simulink model "modelsCompare"  (R2023a)
settings: Solver=ode1  StartTime=0  StopTime=200  FixedStep=0.001  RelTol=1e-3  EnableMultiTasking=on
values from neighbouring files (symbols this model uses):
  B = b*L*(K_v)^2 /J_xx    (= 0.042375883612)    [advanced_model_setup.m]    (also in brusselator.m = 2.15; cycle_detection.m = img2; cycle_detection_start.m = img2; demonstrateDetections.m = 2.15)
  B1 = [-kQ, -kQ, kQ, kQ ... (first row only)    [advanced_model_setup.m]    (also in modelCompPlot.m; set_model_params.m)
  B2 = [0, 0, 0 ... (first row only)    [advanced_model_setup.m]    (also in modelCompPlot.m; set_model_params.m)
  f_p = 1.3    [advanced_model_setup.m]    (also in modelCompPlot.m)
  f_r = 0.4    [advanced_model_setup.m]    (also in modelCompPlot.m)
  f_y = 0.175    [advanced_model_setup.m]    (also in modelCompPlot.m)
  g_p = 10.5    [advanced_model_setup.m]    (also in modelCompPlot.m)
  g_r = 5.2    [advanced_model_setup.m]    (also in modelCompPlot.m)
  I_xx = 0.0522    [advanced_model_setup.m]    (also in modelCompPlot.m; set_model_params.m; solveSyms3d_2.m = evalin('base', 'I_xx'))
  I_yy = 0.0522    [advanced_model_setup.m]    (also in modelCompPlot.m; set_model_params.m; solveSyms3d_2.m = evalin('base', 'I_yy'))
  I_zz = 0.1104    [advanced_model_setup.m]    (also in modelCompPlot.m; set_model_params.m; solveSyms3d_2.m = evalin('base', 'I_zz'))
  J = (J_yy - J_zz)/J_xx    (= -1)    [advanced_model_setup.m]    (also in modelCompPlot.m)
  J_r = J_inertia/J_xx    (= 0.00108695652174)    [advanced_model_setup.m]    (also in modelCompPlot.m; solveSyms3d.m = evalin('base', 'J_r'))
  Jp = 2*Jeq_prop    (= 0.0552224595625)    [modelCompPlot.m]    (also in set_model_params.m)
  Jr = 2*Jeq_prop    (= 0.0552224595625)    [modelCompPlot.m]    (also in set_model_params.m)
  Jy = 4*Jeq_prop    (= 0.110444919125)    [modelCompPlot.m]    (also in set_model_params.m)
  K_v = 54.945    [advanced_model_setup.m]    (also in modelCompPlot.m; solveSyms3d.m = evalin('base', 'K_v'))
  Kf = 0.1188    [modelCompPlot.m]    (also in set_model_params.m)
  kfr_p = 0.4*u2line/x5line    (= 0.285774113641)    [advanced_model_setup.m]    (also in modelCompPlot.m; set_model_params.m)
  kfr_r = 0.4*u1line/x4line    (= 0.285774113641)    [advanced_model_setup.m]    (also in modelCompPlot.m; set_model_params.m)
  kfr_y = 0.4*u3line/x6line    (= 0.0880063173321)    [advanced_model_setup.m]    (also in modelCompPlot.m; set_model_params.m)
  Kt = 0.0036    [modelCompPlot.m]    (also in set_model_params.m)
  L = 0.1969    [advanced_model_setup.m]    (also in modelCompPlot.m; set_model_params.m = 0.19685)
  sigma = 0    [modelCompPlot.m]
  Y = d*(K_v)^2 /J_zz    (= 0.0032609614876)    [advanced_model_setup.m]    (also in modelCompPlot.m; solveSyms3d.m = evalin('base', 'Y'))
libraries: simulink_extras x3, dspsrcs4 x3
settings Model: ExtModeTrigDuration=10000  Creator=kille  LastModifiedBy=Jacob
settings SolverCC: PositivePriorityOrder=on  AutoInsertRateTranBlk=on
settings DataIOCC: ReturnWorkspaceOutputs=off
settings OptimizationCC: LifeSpan=inf
settings DebuggingCC: UnconnectedInputMsg=warning  UnconnectedOutputMsg=warning  UnconnectedLineMsg=warning  ArithmeticOperatorsInVariantConditions=warning
settings ModelReferenceCC: EnableRefExpFcnMdlSchedulingChecks=on
settings SFSimCC: SimUseLocalCustomCode=off  CustomCodeUndefinedFunction=UseInterfaceOnly
settings RTWCC: Description=QUARC Win64 Target  SystemTargetFile=quarc_win64.tlc  TemplateMakefile=quarc_default_tmf  RTWUseLocalCustomCode=off
settings CodeAppCC: StateflowObjectComments=on
settings STFCustomTargetCC: TargetPreCompLibLocation=C:\PROGRA~3\QUARC\lib\2016a\win64\release  UseToolchainInfoCompliant=off  SystemTargetFile=quarc_win64.tlc
settings GRTTargetCC: TargetPreCompLibLocation=C:\PROGRA~3\QUARC\lib\2016a\win64\release  ParMdlRefBuildCompliant=off  CompOptLevelCompliant=off  CombineOutputUpdateFcns=off  MatFileLogging=off  CPPClassGenCompliant=off  GRTInterface=on  UseToolchainInfoCompliant=off  ExtMode=on  ExtModeMexFile=quarc_comm
settings ConfigComp: CovMetricSettings=dswe

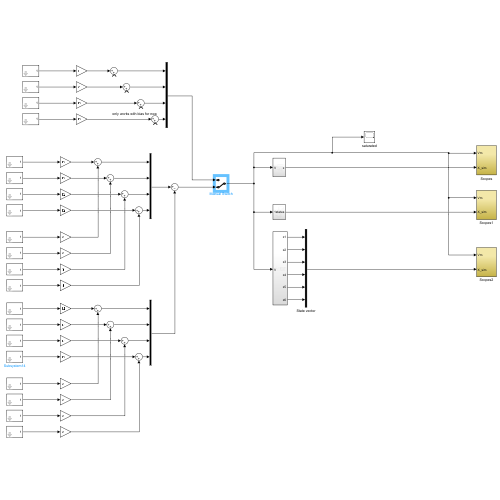
[thumbnail: Simulink's stored preview of the top-level diagram]
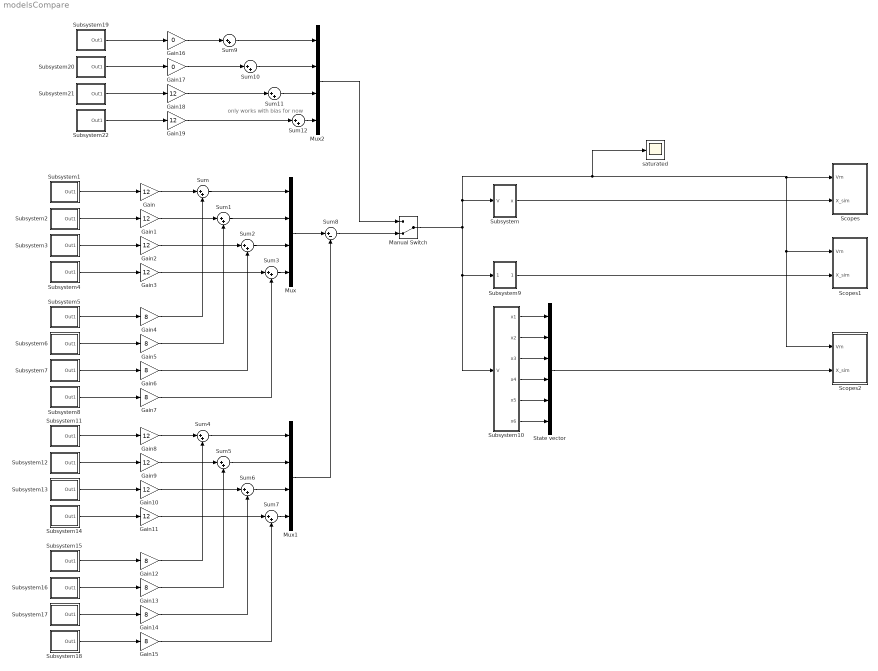
== system modelsCompare ==
  note: only works with bias for now
  Gain{,1..3,8..11,18..19} (10 alike) : Gain  Gain=12
  Gain{4..7,12..15} (8 alike) : Gain  Gain=8
  Gain16 : Gain  Gain=0
  Gain17 : Gain  Gain=0
  Manual Switch : ManualSwitch  CurrentSetting=0
  Mux : Mux
  Mux1 : Mux
  Mux2 : Mux
  Scopes : Subsystem
  Scopes1 : Subsystem
  Scopes2 : Subsystem
  State vector : Mux  Inputs=6
  Subsystem : Subsystem
  Subsystem1 : Subsystem  mask{startTime=15, duration=5, amplitude=1}
      mask prompts: startTime "Start Time"
  Subsystem10 : Subsystem
  Subsystem11 : Subsystem  mask{startTime=215, duration=5, amplitude=1}
      mask prompts: startTime "Start Time"
  Subsystem12 : Subsystem  mask{startTime=260, duration=5, amplitude=1}
      mask prompts: startTime "Start Time"
  Subsystem13 : Subsystem  mask{startTime=305, duration=5, amplitude=1}
      mask prompts: startTime "Start Time"
  Subsystem14 : Subsystem  mask{startTime=350, duration=5, amplitude=1}
      mask prompts: startTime "Start Time"
  Subsystem15 : Subsystem  mask{startTime=240, duration=5, amplitude=1}
      mask prompts: startTime "Start Time"
  Subsystem16 : Subsystem  mask{startTime=285, duration=5, amplitude=1}
      mask prompts: startTime "Start Time"
  Subsystem17 : Subsystem  mask{startTime=330, duration=5, amplitude=1}
      mask prompts: startTime "Start Time"
  Subsystem18 : Subsystem  mask{startTime=375, duration=5, amplitude=1}
      mask prompts: startTime "Start Time"
  Subsystem19 : Subsystem  mask{startTime=15, duration=5, amplitude=1}
      mask prompts: startTime "Start Time"
  Subsystem2 : Subsystem  mask{startTime=60, duration=5, amplitude=1}
      mask prompts: startTime "Start Time"
  Subsystem20 : Subsystem  mask{startTime=60, duration=5, amplitude=1}
      mask prompts: startTime "Start Time"
  Subsystem21 : Subsystem  mask{startTime=105, duration=5, amplitude=1}
      mask prompts: startTime "Start Time"
  Subsystem22 : Subsystem  mask{startTime=150, duration=5, amplitude=1}
      mask prompts: startTime "Start Time"
  Subsystem3 : Subsystem  mask{startTime=105, duration=5, amplitude=1}
      mask prompts: startTime "Start Time"
  Subsystem4 : Subsystem  mask{startTime=150, duration=5, amplitude=1}
      mask prompts: startTime "Start Time"
  Subsystem5 : Subsystem  mask{startTime=40, duration=5, amplitude=1}
      mask prompts: startTime "Start Time"
  Subsystem6 : Subsystem  mask{startTime=85, duration=5, amplitude=1}
      mask prompts: startTime "Start Time"
  Subsystem7 : Subsystem  mask{startTime=130, duration=5, amplitude=1}
      mask prompts: startTime "Start Time"
  Subsystem8 : Subsystem  mask{startTime=175, duration=5, amplitude=1}
      mask prompts: startTime "Start Time"
  Subsystem9 : Subsystem
  Sum{,1..7,9..12} (12 alike) : Sum  Inputs=|++
  Sum8 : Sum  Inputs=|+-
  saturated : Scope
  wires:
  Mux/1 -> Sum8/1
  Sum3/1 -> Mux/4
  Subsystem4/1(Out1) -> Gain3/1
  Subsystem3/1(Out1) -> Gain2/1
  Sum2/1 -> Mux/3
  Subsystem2/1(Out1) -> Gain1/1
  Sum1/1 -> Mux/2
  Subsystem1/1(Out1) -> Gain/1
  Sum/1 -> Mux/1
  Subsystem5/1(Out1) -> Gain4/1
  Subsystem6/1(Out1) -> Gain5/1
  Subsystem7/1(Out1) -> Gain6/1
  Subsystem8/1(Out1) -> Gain7/1
  Subsystem/1(x) -> Scopes/2(X_sim)
  Subsystem10/6(x6) -> State vector/6
  Subsystem10/5(x5) -> State vector/5
  Subsystem10/4(x4) -> State vector/4
  Subsystem10/3(x3) -> State vector/3
  Subsystem10/2(x2) -> State vector/2
  Subsystem10/1(x1) -> State vector/1
  State vector/1 -> Scopes2/2(X_sim)
  Subsystem9/1(states) -> Scopes1/2(X_sim)
  Gain/1 -> Sum/1
  Gain1/1 -> Sum1/1
  Gain2/1 -> Sum2/1
  Gain3/1 -> Sum3/1
  Gain4/1 -> Sum/2
  Gain5/1 -> Sum1/2
  Gain6/1 -> Sum2/2
  Gain7/1 -> Sum3/2
  Subsystem16/1(Out1) -> Gain13/1
  Subsystem14/1(Out1) -> Gain11/1
  Subsystem17/1(Out1) -> Gain14/1
  Subsystem18/1(Out1) -> Gain15/1
  Subsystem15/1(Out1) -> Gain12/1
  Sum5/1 -> Mux1/2
  Gain13/1 -> Sum5/2
  Gain12/1 -> Sum4/2
  Gain10/1 -> Sum6/1
  Subsystem11/1(Out1) -> Gain8/1
  Gain9/1 -> Sum5/1
  Gain11/1 -> Sum7/1
  Gain15/1 -> Sum7/2
  Subsystem13/1(Out1) -> Gain10/1
  Gain14/1 -> Sum6/2
  Sum7/1 -> Mux1/4
  Subsystem12/1(Out1) -> Gain9/1
  Sum4/1 -> Mux1/1
  Gain8/1 -> Sum4/1
  Sum6/1 -> Mux1/3
  Mux1/1 -> Sum8/2
  Manual Switch/1 -> Subsystem9/1(Input), Subsystem10/1(V), saturated/1, Scopes2/1(Vm), Scopes1/1(Vm), Scopes/1(Vm), Subsystem/1(V)
  Sum8/1 -> Manual Switch/2
  Subsystem22/1(Out1) -> Gain19/1
  Sum10/1 -> Mux2/2
  Mux2/1 -> Manual Switch/1
  Gain18/1 -> Sum11/1
  Subsystem19/1(Out1) -> Gain16/1
  Gain17/1 -> Sum10/1
  Gain19/1 -> Sum12/1
  Subsystem21/1(Out1) -> Gain18/1
  Sum12/1 -> Mux2/4
  Subsystem20/1(Out1) -> Gain17/1
  Sum9/1 -> Mux2/1
  Gain16/1 -> Sum9/1
  Sum11/1 -> Mux2/3

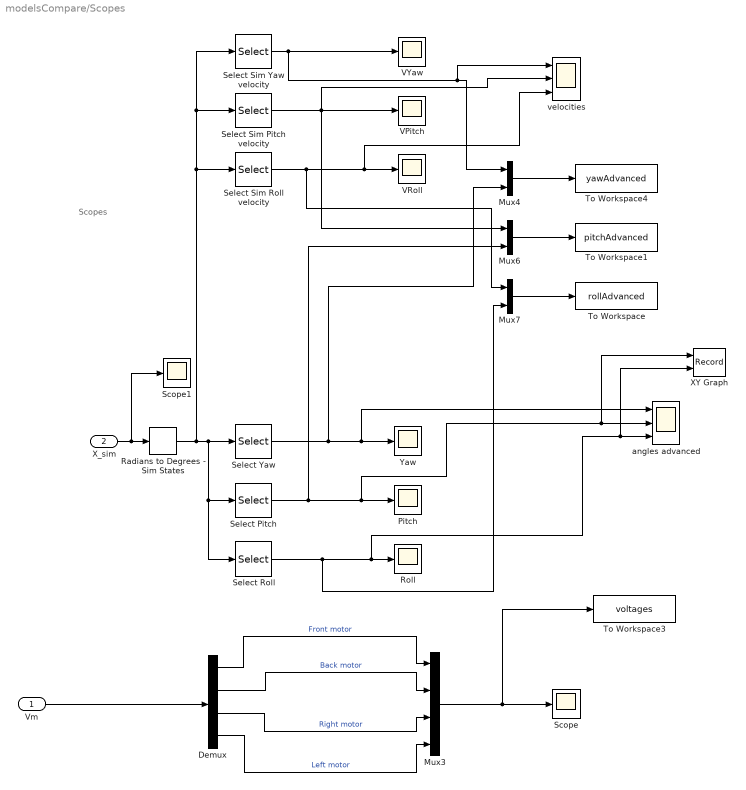
== system modelsCompare/Scopes ==
  note: Scopes
  Vm : Inport
  X_sim : Inport  Port=2
  Demux : Demux
  Mux3 : Mux
  Mux4 : Mux  Inputs=2
  Mux6 : Mux  Inputs=2
  Mux7 : Mux  Inputs=2
  Pitch : Scope
  Radians to Degrees - Sim States : simulink_extras/Transformations/Radians to Degrees
  Roll : Scope
  Scope : Scope
  Scope1 : Scope
  Select Pitch : Selector  InputPortWidth=6  IndexOptions=Index vector (dialog)  Indices=2  OutputSizes=1
  Select Roll : Selector  InputPortWidth=6  IndexOptions=Index vector (dialog)  Indices=3  OutputSizes=1
  Select Sim Pitch velocity : Selector  InputPortWidth=6  IndexOptions=Index vector (dialog)  Indices=5  OutputSizes=1
  Select Sim Roll velocity : Selector  InputPortWidth=6  IndexOptions=Index vector (dialog)  Indices=6  OutputSizes=1
  Select Sim Yaw velocity : Selector  InputPortWidth=6  IndexOptions=Index vector (dialog)  Indices=4  OutputSizes=1
  Select Yaw : Selector  InputPortWidth=6  IndexOptions=Index vector (dialog)  Indices=1  OutputSizes=1
  To Workspace : ToWorkspace  VariableName=rollAdvanced  SampleTime=-1
  To Workspace1 : ToWorkspace  VariableName=pitchAdvanced  SampleTime=-1
  To Workspace3 : ToWorkspace  VariableName=voltages  SampleTime=-1
  To Workspace4 : ToWorkspace  VariableName=yawAdvanced  SampleTime=-1
  VPitch : Scope
  VRoll : Scope
  VYaw : Scope
  XY Graph : Record  FileSettingsInternal="{\"entries\":[{\"content\":{\"excelSettings\":{\"content\":{},\"type\":\"Streamout.ExcelSettings\"}},\"type\":\"Streamout.FileSettingStorage\",\"uuid\":\"\"}],\"packageUris\":[\"http:\\/\\/schema.mathworks.com\\/mf0\\/streamout_blocks\\/R2020a\"],\"version\":\"1.0\"}"  Layout=[1 1]  SignalsInternal="{\"entries\":[{\"content\":{\"signals\":[{\"content\":{\"blockPath\":[],\"dimensions\":[1],\"domain\":\"\",\"lineColor\":\"#d95319\",\"port\":1,\"sid\":[\"\"],\"signalID\":2812,\"signalName\":\"Select Pitch\"},\"type\":\"RecordBlkView.Signal\",\"uuid\":\"\"},{\"content\":{\"blockPath\":[],\"dimensions\":[1],\"domain\":\"\",\"lineColor\":\"#edb120\",\"port\":2,\"sid\":[\"\"],\"signalID\":2816,\"signalName\":\"Select Roll\"},\"type\":\"RecordBlkView.Signal\",\"uuid\":\"\"}]},\"type\":\"RecordBlkView.InputSignals\",\"uuid\":\"\"}],\"packageUris\":[\"http:\\/\\/schema.mathworks.com\\/mf0\\/streamout_blocks\\/R2020a\"],\"version\":\"1.0\"}"  VisualizationBindings="{\"xyplotplugin\":{\"info\":[{\"series\":[],\"subplotID\":1}]}}"  CompatibilityTag=XY
  Yaw : Scope
  angles advanced : Scope  NumInputPorts=3
  velocities : Scope  NumInputPorts=3
  wires:
  Select Roll/1 -> XY Graph/2, angles advanced/3, Roll/1, Mux7/2
  Radians to Degrees - Sim States/1 -> Select Sim Roll velocity/1, Select Sim Pitch velocity/1, Select Sim Yaw velocity/1, Select Roll/1, Select Pitch/1, Select Yaw/1
  Select Pitch/1 -> XY Graph/1, angles advanced/2, Pitch/1, Mux6/2
  X_sim/1 -> Scope1/1, Radians to Degrees - Sim States/1
  Demux/1 -> Mux3/1  "Front motor"
  Demux/2 -> Mux3/2  "Back motor"
  Demux/3 -> Mux3/3  "Right motor"
  Demux/4 -> Mux3/4  "Left motor"
  Vm/1 -> Demux/1
  Select Sim Yaw velocity/1 -> VYaw/1, velocities/1, Mux4/1
  Select Sim Roll velocity/1 -> velocities/3, VRoll/1, Mux7/1
  Select Sim Pitch velocity/1 -> Mux6/1, velocities/2, VPitch/1
  Mux4/1 -> To Workspace4/1
  Mux6/1 -> To Workspace1/1
  Mux7/1 -> To Workspace/1
  Mux3/1 -> To Workspace3/1, Scope/1
  Select Yaw/1 -> angles advanced/1, Yaw/1, Mux4/2

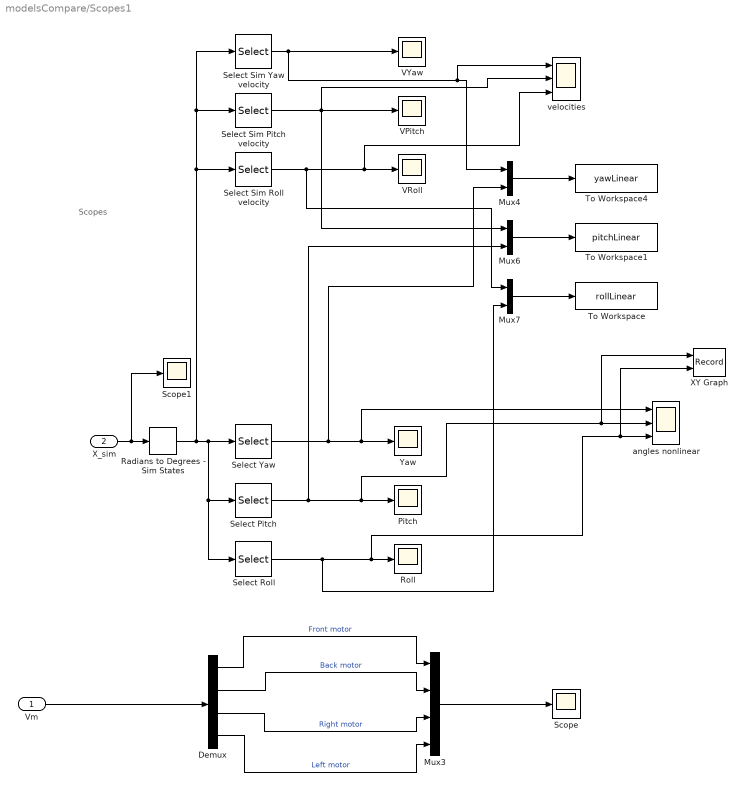
== system modelsCompare/Scopes1 ==
  note: Scopes
  Vm : Inport
  X_sim : Inport  Port=2
  Demux : Demux
  Mux3 : Mux
  Mux4 : Mux  Inputs=2
  Mux6 : Mux  Inputs=2
  Mux7 : Mux  Inputs=2
  Pitch : Scope
  Radians to Degrees - Sim States : simulink_extras/Transformations/Radians to Degrees
  Roll : Scope
  Scope : Scope
  Scope1 : Scope
  Select Pitch : Selector  InputPortWidth=6  IndexOptions=Index vector (dialog)  Indices=2  OutputSizes=1
  Select Roll : Selector  InputPortWidth=6  IndexOptions=Index vector (dialog)  Indices=3  OutputSizes=1
  Select Sim Pitch velocity : Selector  InputPortWidth=6  IndexOptions=Index vector (dialog)  Indices=5  OutputSizes=1
  Select Sim Roll velocity : Selector  InputPortWidth=6  IndexOptions=Index vector (dialog)  Indices=6  OutputSizes=1
  Select Sim Yaw velocity : Selector  InputPortWidth=6  IndexOptions=Index vector (dialog)  Indices=4  OutputSizes=1
  Select Yaw : Selector  InputPortWidth=6  IndexOptions=Index vector (dialog)  Indices=1  OutputSizes=1
  To Workspace : ToWorkspace  VariableName=rollLinear  SampleTime=-1
  To Workspace1 : ToWorkspace  VariableName=pitchLinear  SampleTime=-1
  To Workspace4 : ToWorkspace  VariableName=yawLinear  SampleTime=-1
  VPitch : Scope
  VRoll : Scope
  VYaw : Scope
  XY Graph : Record  FileSettingsInternal="{\"entries\":[{\"content\":{\"excelSettings\":{\"content\":{},\"type\":\"Streamout.ExcelSettings\"}},\"type\":\"Streamout.FileSettingStorage\",\"uuid\":\"\"}],\"packageUris\":[\"http:\\/\\/schema.mathworks.com\\/mf0\\/streamout_blocks\\/R2020a\"],\"version\":\"1.0\"}"  Layout=[1 1]  SignalsInternal="{\"entries\":[{\"content\":{\"signals\":[{\"content\":{\"blockPath\":[],\"dimensions\":[1],\"domain\":\"\",\"lineColor\":\"#b746ff\",\"port\":1,\"sid\":[\"\"],\"signalID\":2835,\"signalName\":\"Select Pitch\"},\"type\":\"RecordBlkView.Signal\",\"uuid\":\"\"},{\"content\":{\"blockPath\":[],\"dimensions\":[1],\"domain\":\"\",\"lineColor\":\"#64d413\",\"port\":2,\"sid\":[\"\"],\"signalID\":2839,\"signalName\":\"Select Roll\"},\"type\":\"RecordBlkView.Signal\",\"uuid\":\"\"}]},\"type\":\"RecordBlkView.InputSignals\",\"uuid\":\"\"}],\"packageUris\":[\"http:\\/\\/schema.mathworks.com\\/mf0\\/streamout_blocks\\/R2020a\"],\"version\":\"1.0\"}"  VisualizationBindings="{\"xyplotplugin\":{\"info\":[{\"series\":[],\"subplotID\":1}]}}"  CompatibilityTag=XY
  Yaw : Scope
  angles nonlinear : Scope  NumInputPorts=3
  velocities : Scope  NumInputPorts=3
  wires:
  Select Roll/1 -> XY Graph/2, angles nonlinear/3, Roll/1, Mux7/2
  Radians to Degrees - Sim States/1 -> Select Sim Roll velocity/1, Select Sim Pitch velocity/1, Select Sim Yaw velocity/1, Select Roll/1, Select Pitch/1, Select Yaw/1
  Select Pitch/1 -> XY Graph/1, angles nonlinear/2, Pitch/1, Mux6/2
  X_sim/1 -> Scope1/1, Radians to Degrees - Sim States/1
  Demux/1 -> Mux3/1  "Front motor"
  Demux/2 -> Mux3/2  "Back motor"
  Demux/3 -> Mux3/3  "Right motor"
  Demux/4 -> Mux3/4  "Left motor"
  Vm/1 -> Demux/1
  Select Sim Yaw velocity/1 -> VYaw/1, velocities/1, Mux4/1
  Select Sim Roll velocity/1 -> velocities/3, VRoll/1, Mux7/1
  Select Sim Pitch velocity/1 -> Mux6/1, velocities/2, VPitch/1
  Mux4/1 -> To Workspace4/1
  Mux6/1 -> To Workspace1/1
  Mux7/1 -> To Workspace/1
  Mux3/1 -> Scope/1
  Select Yaw/1 -> angles nonlinear/1, Yaw/1, Mux4/2

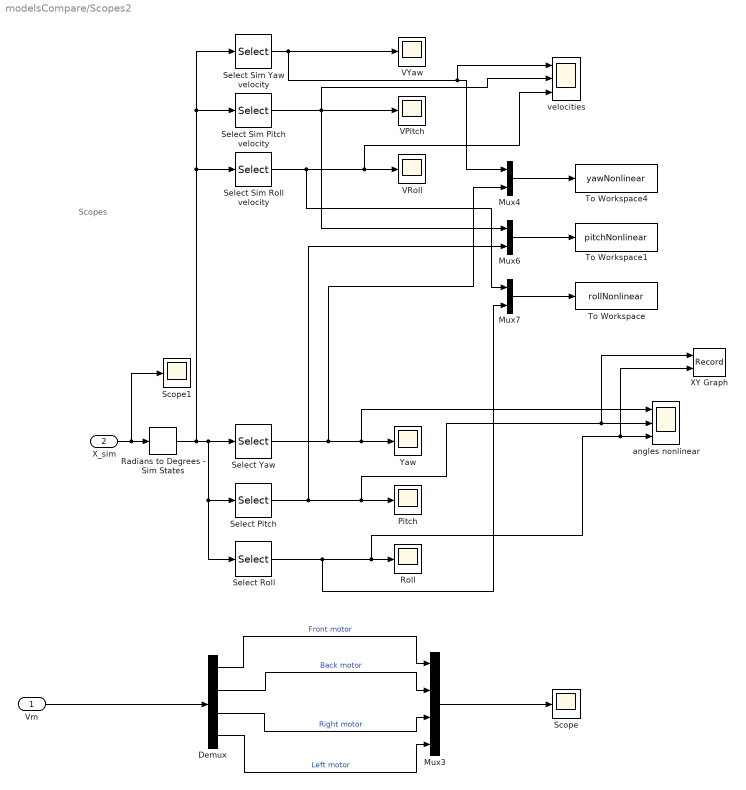
== system modelsCompare/Scopes2 ==
  note: Scopes
  Vm : Inport
  X_sim : Inport  Port=2
  Demux : Demux
  Mux3 : Mux
  Mux4 : Mux  Inputs=2
  Mux6 : Mux  Inputs=2
  Mux7 : Mux  Inputs=2
  Pitch : Scope
  Radians to Degrees - Sim States : simulink_extras/Transformations/Radians to Degrees
  Roll : Scope
  Scope : Scope
  Scope1 : Scope
  Select Pitch : Selector  InputPortWidth=6  IndexOptions=Index vector (dialog)  Indices=2  OutputSizes=1
  Select Roll : Selector  InputPortWidth=6  IndexOptions=Index vector (dialog)  Indices=3  OutputSizes=1
  Select Sim Pitch velocity : Selector  InputPortWidth=6  IndexOptions=Index vector (dialog)  Indices=5  OutputSizes=1
  Select Sim Roll velocity : Selector  InputPortWidth=6  IndexOptions=Index vector (dialog)  Indices=6  OutputSizes=1
  Select Sim Yaw velocity : Selector  InputPortWidth=6  IndexOptions=Index vector (dialog)  Indices=4  OutputSizes=1
  Select Yaw : Selector  InputPortWidth=6  IndexOptions=Index vector (dialog)  Indices=1  OutputSizes=1
  To Workspace : ToWorkspace  VariableName=rollNonlinear  SampleTime=-1
  To Workspace1 : ToWorkspace  VariableName=pitchNonlinear  SampleTime=-1
  To Workspace4 : ToWorkspace  VariableName=yawNonlinear  SampleTime=-1
  VPitch : Scope
  VRoll : Scope
  VYaw : Scope
  XY Graph : Record  FileSettingsInternal="{\"entries\":[{\"content\":{\"excelSettings\":{\"content\":{},\"type\":\"Streamout.ExcelSettings\"}},\"type\":\"Streamout.FileSettingStorage\",\"uuid\":\"\"}],\"packageUris\":[\"http:\\/\\/schema.mathworks.com\\/mf0\\/streamout_blocks\\/R2020a\"],\"version\":\"1.0\"}"  Layout=[1 1]  SignalsInternal="{\"entries\":[{\"content\":{\"signals\":[{\"content\":{\"blockPath\":[],\"dimensions\":[1],\"domain\":\"\",\"lineColor\":\"#7e2f8e\",\"port\":1,\"sid\":[\"\"],\"signalID\":2858,\"signalName\":\"Select Pitch\"},\"type\":\"RecordBlkView.Signal\",\"uuid\":\"\"},{\"content\":{\"blockPath\":[],\"dimensions\":[1],\"domain\":\"\",\"lineColor\":\"#77ac30\",\"port\":2,\"sid\":[\"\"],\"signalID\":2862,\"signalName\":\"Select Roll\"},\"type\":\"RecordBlkView.Signal\",\"uuid\":\"\"}]},\"type\":\"RecordBlkView.InputSignals\",\"uuid\":\"\"}],\"packageUris\":[\"http:\\/\\/schema.mathworks.com\\/mf0\\/streamout_blocks\\/R2020a\"],\"version\":\"1.0\"}"  VisualizationBindings="{\"xyplotplugin\":{\"info\":[{\"series\":[],\"subplotID\":1}]}}"  CompatibilityTag=XY
  Yaw : Scope
  angles nonlinear : Scope  NumInputPorts=3
  velocities : Scope  NumInputPorts=3
  wires:
  Select Roll/1 -> XY Graph/2, angles nonlinear/3, Roll/1, Mux7/2
  Radians to Degrees - Sim States/1 -> Select Sim Roll velocity/1, Select Sim Pitch velocity/1, Select Sim Yaw velocity/1, Select Roll/1, Select Pitch/1, Select Yaw/1
  Select Pitch/1 -> XY Graph/1, angles nonlinear/2, Pitch/1, Mux6/2
  X_sim/1 -> Scope1/1, Radians to Degrees - Sim States/1
  Demux/1 -> Mux3/1  "Front motor"
  Demux/2 -> Mux3/2  "Back motor"
  Demux/3 -> Mux3/3  "Right motor"
  Demux/4 -> Mux3/4  "Left motor"
  Vm/1 -> Demux/1
  Select Sim Yaw velocity/1 -> VYaw/1, velocities/1, Mux4/1
  Select Sim Roll velocity/1 -> velocities/3, VRoll/1, Mux7/1
  Select Sim Pitch velocity/1 -> Mux6/1, velocities/2, VPitch/1
  Mux4/1 -> To Workspace4/1
  Mux6/1 -> To Workspace1/1
  Mux7/1 -> To Workspace/1
  Mux3/1 -> Scope/1
  Select Yaw/1 -> angles nonlinear/1, Yaw/1, Mux4/2

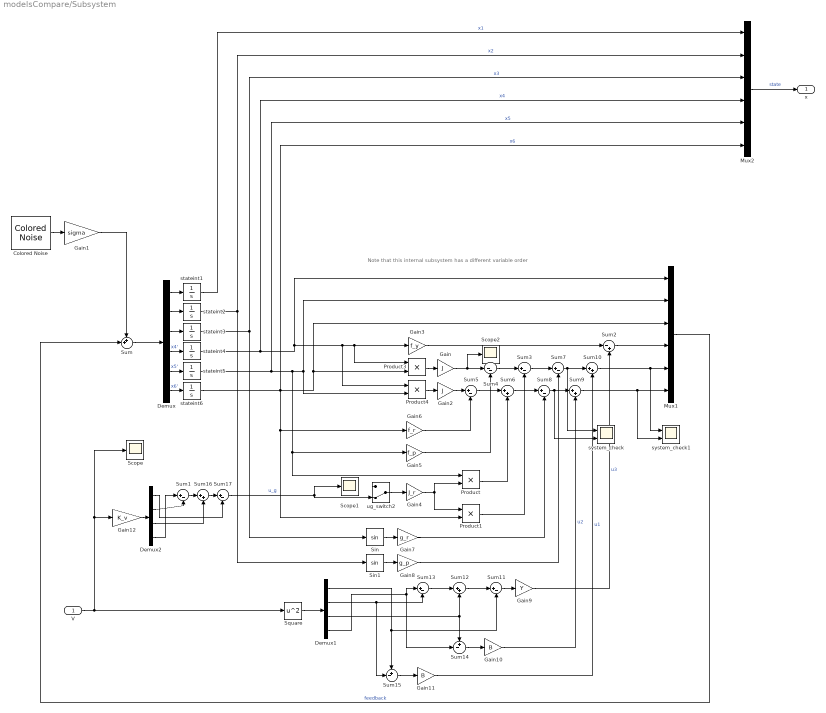
== system modelsCompare/Subsystem ==
  note: Note that this internal subsystem has a different variable order
  V : Inport
  Colored Noise : dspsrcs4/Colored Noise  Color=white  InverseFrequencyPower=1  BoundedOutput=off  NumChannels=6  OutputDataType=double  SamplesPerFrame=1  SampleTime=1  RandomStream=mt19937ar with seed  Seed=67  SimulateUsing=Interpreted execution
  Demux : Demux  Outputs=6
  Demux1 : Demux
  Demux2 : Demux
  Gain : Gain  Gain=J
  Gain1 : Gain  Gain=sigma
  Gain10 : Gain  Gain=B
  Gain11 : Gain  Gain=B
  Gain12 : Gain  Gain=K_v
  Gain2 : Gain  Gain=J
  Gain3 : Gain  Gain=f_y
  Gain4 : Gain  Gain=J_r
  Gain5 : Gain  Gain=f_p
  Gain6 : Gain  Gain=f_r
  Gain7 : Gain  Gain=g_r
  Gain8 : Gain  Gain=g_p
  Gain9 : Gain  Gain=Y
  Mux1 : Mux  Inputs=6
  Mux2 : Mux  Inputs=6
  Product{,1,3..4} (4 alike) : Product
  Scope : Scope
  Scope1 : Scope
  Scope2 : Scope
  Sin : Trigonometry
  Sin1 : Trigonometry
  Square : Math  Operator=square
  Sum : Sum  Inputs=++|
  Sum{1,3,5,7..8,11,13,17} (8 alike) : Sum  Inputs=|+-
  Sum{6,9..10,12,16} (5 alike) : Sum  Inputs=|++
  Sum14 : Sum  Inputs=+-|
  Sum15 : Sum  Inputs=+-|
  Sum2 : Sum  Inputs=|-+
  Sum4 : Sum  Inputs=|--
  stateint{1..6} (6 alike) : Integrator
  system_check : Scope  NumInputPorts=2
  system_check1 : Scope  NumInputPorts=2
  ug_switch2 : ManualSwitch  CurrentSetting=0
  x : Outport
  wires:
  stateint5/1 -> Mux2/5, Gain5/1, Product/1, Product4/2, Mux1/2  "x5"
  stateint4/1 -> Mux2/4, Mux1/1, Product4/1, Product3/1, Gain3/1  "x4"
  Demux/1 -> stateint1/1
  stateint6/1 -> Mux2/6, Gain6/1, Product1/2, Product3/2, Mux1/3  "x6"
  Demux/6 -> stateint6/1  "x6'"
  Demux/5 -> stateint5/1  "x5'"
  Demux/2 -> stateint2/1
  Demux/3 -> stateint3/1
  Demux/4 -> stateint4/1  "x4'"
  Product3/1 -> Gain/1
  Product4/1 -> Gain2/1
  Colored Noise/1 -> Gain1/1
  Sum/1 -> Demux/1
  Gain1/1 -> Sum/1
  Gain3/1 -> Sum2/1
  Gain4/1 -> Product1/1, Product/2
  Sum17/1 -> ug_switch2/2, Scope1/1  "u_g"
  Gain/1 -> Scope2/1, Sum4/1
  Gain2/1 -> Sum5/1
  Gain6/1 -> Sum5/2
  Gain5/1 -> Sum4/2
  Sum5/1 -> Sum6/1
  Product/1 -> Sum6/2
  Sum4/1 -> Sum3/1
  Sum6/1 -> Sum8/1
  Sum3/1 -> Sum7/1
  Gain7/1 -> Sum8/2
  Gain8/1 -> Sum7/2
  Sin/1 -> Gain7/1
  Sin1/1 -> Gain8/1
  Sum8/1 -> system_check/2, Sum9/1
  Sum7/1 -> system_check/1, Sum10/1
  Sum11/1 -> Gain9/1
  Gain9/1 -> Sum2/2  "u3"
  Square/1 -> Demux1/1
  Sum12/1 -> Sum11/1
  Sum13/1 -> Sum12/1
  Demux1/4 -> Sum13/1, Sum14/2
  Demux1/2 -> Sum13/2, Sum15/2
  Demux1/3 -> Sum12/2, Sum14/1
  Demux1/1 -> Sum15/1, Sum11/2
  Sum14/1 -> Gain10/1
  Sum15/1 -> Gain11/1
  Gain10/1 -> Sum9/2  "u2"
  Gain11/1 -> Sum10/2  "u1"
  Mux1/1 -> Sum/2  "feedback"
  V/1 -> Square/1, Scope/1, Gain12/1
  Gain12/1 -> Demux2/1
  Sum1/1 -> Sum16/1
  Sum16/1 -> Sum17/1
  Demux2/2 -> Sum1/2
  Demux2/3 -> Sum16/2
  Sum10/1 -> system_check1/1, Mux1/5
  Sum2/1 -> Mux1/4
  stateint2/1 -> Mux2/2, Sin1/1  "x2"
  stateint3/1 -> Mux2/3, Sin/1  "x3"
  Product1/1 -> Sum3/2
  Demux2/4 -> Sum1/1
  Demux2/1 -> Sum17/2
  stateint1/1 -> Mux2/1  "x1"
  Mux2/1 -> x/1  "state"
  Sum9/1 -> system_check1/2, Mux1/6
  ug_switch2/1 -> Gain4/1

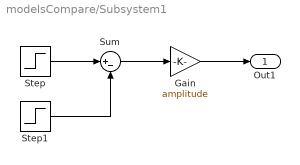
== system modelsCompare/Subsystem1 ==
  Gain : Gain  Gain=amplitude
  Step : Step  Time=startTime  SampleTime=0
  Step1 : Step  Time=startTime+duration  SampleTime=0
  Sum : Sum  Inputs=|+-
  Out1 : Outport
  wires:
  Sum/1 -> Gain/1
  Step/1 -> Sum/1
  Gain/1 -> Out1/1
  Step1/1 -> Sum/2

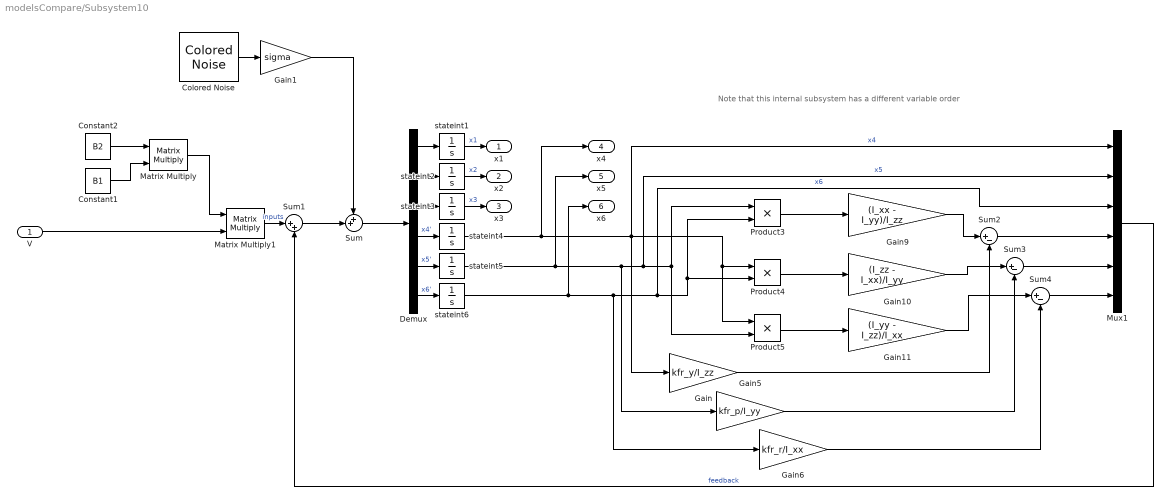
== system modelsCompare/Subsystem10 ==
  note: Note that this internal subsystem has a different variable order
  V : Inport
  Colored Noise : dspsrcs4/Colored Noise  Color=white  InverseFrequencyPower=1  BoundedOutput=off  NumChannels=6  OutputDataType=double  SamplesPerFrame=1  SampleTime=1  RandomStream=mt19937ar with seed  Seed=67  SimulateUsing=Interpreted execution
  Constant1 : Constant  Value=B1
  Constant2 : Constant  Value=B2
  Demux : Demux  Outputs=6
  Gain : Gain  Gain=kfr_y/I_zz
  Gain1 : Gain  Gain=sigma
  Gain10 : Gain  Gain=(I_zz - I_xx)/I_yy
  Gain11 : Gain  Gain=(I_yy - I_zz)/I_xx
  Gain5 : Gain  Gain=kfr_p/I_yy
  Gain6 : Gain  Gain=kfr_r/I_xx
  Gain9 : Gain  Gain=(I_xx - I_yy)/I_zz
  Matrix Multiply : Product  Multiplication=Matrix(*)
  Matrix Multiply1 : Product  Multiplication=Matrix(*)
  Mux1 : Mux  Inputs=6
  Product3 : Product
  Product4 : Product
  Product5 : Product
  Sum : Sum  Inputs=++|
  Sum1 : Sum  Inputs=|++
  Sum2 : Sum  Inputs=|+-
  Sum3 : Sum  Inputs=|+-
  Sum4 : Sum  Inputs=|+-
  stateint{1..6} (6 alike) : Integrator
  x1 : Outport
  x2 : Outport  Port=2
  x3 : Outport  Port=3
  x4 : Outport  Port=4
  x5 : Outport  Port=5
  x6 : Outport  Port=6
  wires:
  Mux1/1 -> Sum1/2  "feedback"
  stateint5/1 -> x5/1, Gain5/1, Mux1/2, Product5/2, Product3/1  "x5"
  Matrix Multiply1/1 -> Sum1/1  "inputs"
  stateint4/1 -> x4/1, Gain/1, Mux1/1, Product5/1, Product4/1  "x4"
  Matrix Multiply/1 -> Matrix Multiply1/1
  V/1 -> Matrix Multiply1/2
  Sum2/1 -> Mux1/4
  Gain6/1 -> Sum4/2
  Demux/1 -> stateint1/1
  stateint6/1 -> x6/1, Gain6/1, Mux1/3, Product4/2, Product3/2  "x6"
  Demux/6 -> stateint6/1  "x6'"
  Product5/1 -> Gain11/1
  Demux/5 -> stateint5/1  "x5'"
  Demux/2 -> stateint2/1
  Gain11/1 -> Sum4/1
  Constant1/1 -> Matrix Multiply/2
  Demux/3 -> stateint3/1
  Gain9/1 -> Sum2/1
  Gain10/1 -> Sum3/1
  Constant2/1 -> Matrix Multiply/1
  Demux/4 -> stateint4/1  "x4'"
  Product4/1 -> Gain10/1
  stateint1/1 -> x1/1  "x1"
  stateint2/1 -> x2/1  "x2"
  stateint3/1 -> x3/1  "x3"
  Colored Noise/1 -> Gain1/1
  Sum1/1 -> Sum/2
  Sum/1 -> Demux/1
  Gain1/1 -> Sum/1
  Product3/1 -> Gain9/1
  Gain/1 -> Sum2/2
  Gain5/1 -> Sum3/2
  Sum4/1 -> Mux1/6
  Sum3/1 -> Mux1/5

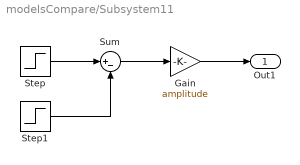
== system modelsCompare/Subsystem11 ==
  Gain : Gain  Gain=amplitude
  Step : Step  Time=startTime  SampleTime=0
  Step1 : Step  Time=startTime+duration  SampleTime=0
  Sum : Sum  Inputs=|+-
  Out1 : Outport
  wires:
  Sum/1 -> Gain/1
  Step/1 -> Sum/1
  Gain/1 -> Out1/1
  Step1/1 -> Sum/2

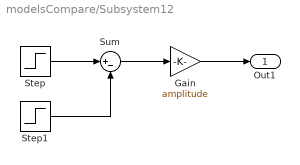
== system modelsCompare/Subsystem12 ==
  Gain : Gain  Gain=amplitude
  Step : Step  Time=startTime  SampleTime=0
  Step1 : Step  Time=startTime+duration  SampleTime=0
  Sum : Sum  Inputs=|+-
  Out1 : Outport
  wires:
  Sum/1 -> Gain/1
  Step/1 -> Sum/1
  Gain/1 -> Out1/1
  Step1/1 -> Sum/2

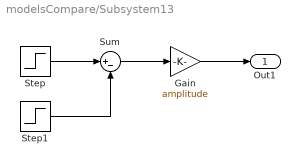
== system modelsCompare/Subsystem13 ==
  Gain : Gain  Gain=amplitude
  Step : Step  Time=startTime  SampleTime=0
  Step1 : Step  Time=startTime+duration  SampleTime=0
  Sum : Sum  Inputs=|+-
  Out1 : Outport
  wires:
  Sum/1 -> Gain/1
  Step/1 -> Sum/1
  Gain/1 -> Out1/1
  Step1/1 -> Sum/2

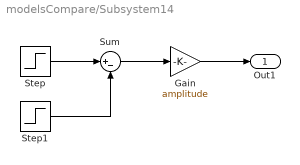
== system modelsCompare/Subsystem14 ==
  Gain : Gain  Gain=amplitude
  Step : Step  Time=startTime  SampleTime=0
  Step1 : Step  Time=startTime+duration  SampleTime=0
  Sum : Sum  Inputs=|+-
  Out1 : Outport
  wires:
  Sum/1 -> Gain/1
  Step/1 -> Sum/1
  Gain/1 -> Out1/1
  Step1/1 -> Sum/2

== system modelsCompare/Subsystem15 ==
  Gain : Gain  Gain=amplitude
  Step : Step  Time=startTime  SampleTime=0
  Step1 : Step  Time=startTime+duration  SampleTime=0
  Sum : Sum  Inputs=|+-
  Out1 : Outport
  wires:
  Sum/1 -> Gain/1
  Step/1 -> Sum/1
  Gain/1 -> Out1/1
  Step1/1 -> Sum/2

== system modelsCompare/Subsystem16 ==
  Gain : Gain  Gain=amplitude
  Step : Step  Time=startTime  SampleTime=0
  Step1 : Step  Time=startTime+duration  SampleTime=0
  Sum : Sum  Inputs=|+-
  Out1 : Outport
  wires:
  Sum/1 -> Gain/1
  Step/1 -> Sum/1
  Gain/1 -> Out1/1
  Step1/1 -> Sum/2

== system modelsCompare/Subsystem17 ==
  Gain : Gain  Gain=amplitude
  Step : Step  Time=startTime  SampleTime=0
  Step1 : Step  Time=startTime+duration  SampleTime=0
  Sum : Sum  Inputs=|+-
  Out1 : Outport
  wires:
  Sum/1 -> Gain/1
  Step/1 -> Sum/1
  Gain/1 -> Out1/1
  Step1/1 -> Sum/2

== system modelsCompare/Subsystem18 ==
  Gain : Gain  Gain=amplitude
  Step : Step  Time=startTime  SampleTime=0
  Step1 : Step  Time=startTime+duration  SampleTime=0
  Sum : Sum  Inputs=|+-
  Out1 : Outport
  wires:
  Sum/1 -> Gain/1
  Step/1 -> Sum/1
  Gain/1 -> Out1/1
  Step1/1 -> Sum/2

== system modelsCompare/Subsystem19 ==
  Gain : Gain  Gain=amplitude
  Step : Step  Time=startTime  SampleTime=0
  Step1 : Step  Time=startTime+duration  SampleTime=0
  Sum : Sum  Inputs=|+-
  Out1 : Outport
  wires:
  Sum/1 -> Gain/1
  Step/1 -> Sum/1
  Gain/1 -> Out1/1
  Step1/1 -> Sum/2

== system modelsCompare/Subsystem2 ==
  Gain : Gain  Gain=amplitude
  Step : Step  Time=startTime  SampleTime=0
  Step1 : Step  Time=startTime+duration  SampleTime=0
  Sum : Sum  Inputs=|+-
  Out1 : Outport
  wires:
  Sum/1 -> Gain/1
  Step/1 -> Sum/1
  Gain/1 -> Out1/1
  Step1/1 -> Sum/2

== system modelsCompare/Subsystem20 ==
  Gain : Gain  Gain=amplitude
  Step : Step  Time=startTime  SampleTime=0
  Step1 : Step  Time=startTime+duration  SampleTime=0
  Sum : Sum  Inputs=|+-
  Out1 : Outport
  wires:
  Sum/1 -> Gain/1
  Step/1 -> Sum/1
  Gain/1 -> Out1/1
  Step1/1 -> Sum/2

== system modelsCompare/Subsystem21 ==
  Gain : Gain  Gain=amplitude
  Step : Step  Time=startTime  SampleTime=0
  Step1 : Step  Time=startTime+duration  SampleTime=0
  Sum : Sum  Inputs=|+-
  Out1 : Outport
  wires:
  Sum/1 -> Gain/1
  Step/1 -> Sum/1
  Gain/1 -> Out1/1
  Step1/1 -> Sum/2

== system modelsCompare/Subsystem22 ==
  Gain : Gain  Gain=amplitude
  Step : Step  Time=startTime  SampleTime=0
  Step1 : Step  Time=startTime+duration  SampleTime=0
  Sum : Sum  Inputs=|+-
  Out1 : Outport
  wires:
  Sum/1 -> Gain/1
  Step/1 -> Sum/1
  Gain/1 -> Out1/1
  Step1/1 -> Sum/2

== system modelsCompare/Subsystem3 ==
  Gain : Gain  Gain=amplitude
  Step : Step  Time=startTime  SampleTime=0
  Step1 : Step  Time=startTime+duration  SampleTime=0
  Sum : Sum  Inputs=|+-
  Out1 : Outport
  wires:
  Sum/1 -> Gain/1
  Step/1 -> Sum/1
  Gain/1 -> Out1/1
  Step1/1 -> Sum/2

== system modelsCompare/Subsystem4 ==
  Gain : Gain  Gain=amplitude
  Step : Step  Time=startTime  SampleTime=0
  Step1 : Step  Time=startTime+duration  SampleTime=0
  Sum : Sum  Inputs=|+-
  Out1 : Outport
  wires:
  Sum/1 -> Gain/1
  Step/1 -> Sum/1
  Gain/1 -> Out1/1
  Step1/1 -> Sum/2

== system modelsCompare/Subsystem5 ==
  Gain : Gain  Gain=amplitude
  Step : Step  Time=startTime  SampleTime=0
  Step1 : Step  Time=startTime+duration  SampleTime=0
  Sum : Sum  Inputs=|+-
  Out1 : Outport
  wires:
  Sum/1 -> Gain/1
  Step/1 -> Sum/1
  Gain/1 -> Out1/1
  Step1/1 -> Sum/2

== system modelsCompare/Subsystem6 ==
  Gain : Gain  Gain=amplitude
  Step : Step  Time=startTime  SampleTime=0
  Step1 : Step  Time=startTime+duration  SampleTime=0
  Sum : Sum  Inputs=|+-
  Out1 : Outport
  wires:
  Sum/1 -> Gain/1
  Step/1 -> Sum/1
  Gain/1 -> Out1/1
  Step1/1 -> Sum/2

== system modelsCompare/Subsystem7 ==
  Gain : Gain  Gain=amplitude
  Step : Step  Time=startTime  SampleTime=0
  Step1 : Step  Time=startTime+duration  SampleTime=0
  Sum : Sum  Inputs=|+-
  Out1 : Outport
  wires:
  Sum/1 -> Gain/1
  Step/1 -> Sum/1
  Gain/1 -> Out1/1
  Step1/1 -> Sum/2

== system modelsCompare/Subsystem8 ==
  Gain : Gain  Gain=amplitude
  Step : Step  Time=startTime  SampleTime=0
  Step1 : Step  Time=startTime+duration  SampleTime=0
  Sum : Sum  Inputs=|+-
  Out1 : Outport
  wires:
  Sum/1 -> Gain/1
  Step/1 -> Sum/1
  Gain/1 -> Out1/1
  Step1/1 -> Sum/2

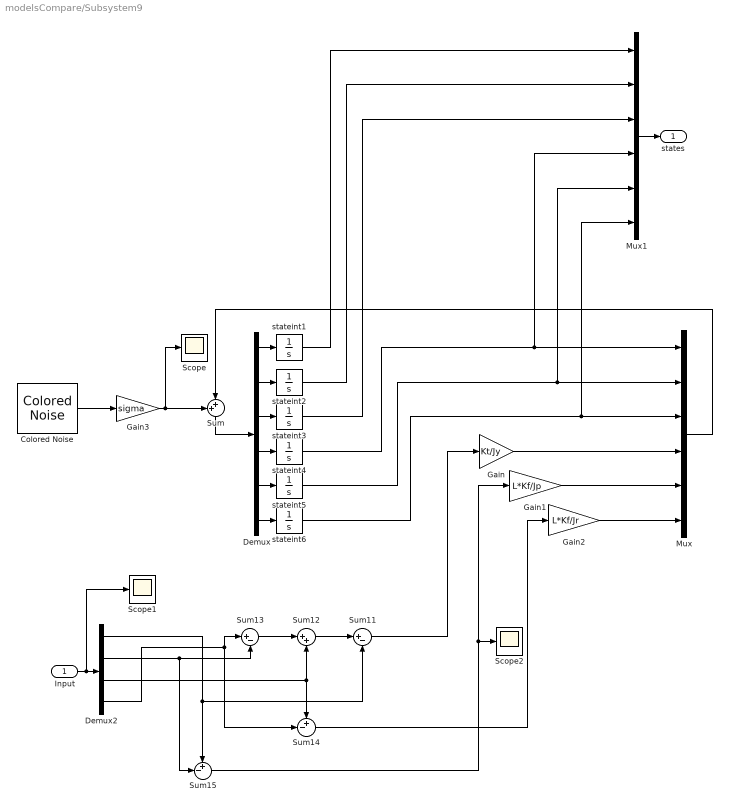
== system modelsCompare/Subsystem9 ==
  Input : Inport
  Colored Noise : dspsrcs4/Colored Noise  Color=white  InverseFrequencyPower=1  BoundedOutput=off  NumChannels=6  OutputDataType=double  SamplesPerFrame=1  SampleTime=1  RandomStream=mt19937ar with seed  Seed=67  SimulateUsing=Interpreted execution
  Demux : Demux  Outputs=6
  Demux2 : Demux
  Gain : Gain  Gain=Kt/Jy
  Gain1 : Gain  Gain=L*Kf/Jp
  Gain2 : Gain  Gain=L*Kf/Jr
  Gain3 : Gain  Gain=sigma
  Mux : Mux  Inputs=6
  Mux1 : Mux  Inputs=6
  Scope : Scope
  Scope1 : Scope
  Scope2 : Scope
  Sum : Sum  Inputs=++|
  Sum11 : Sum  Inputs=|+-
  Sum12 : Sum  Inputs=|++
  Sum13 : Sum  Inputs=|+-
  Sum14 : Sum  Inputs=+-|
  Sum15 : Sum  Inputs=+-|
  stateint{1..6} (6 alike) : Integrator
  states : Outport
  wires:
  stateint5/1 -> Mux/2, Mux1/5
  Gain2/1 -> Mux/6
  Gain1/1 -> Mux/5
  stateint6/1 -> Mux/3, Mux1/6
  stateint4/1 -> Mux/1, Mux1/4
  Gain/1 -> Mux/4
  Mux/1 -> Sum/2
  Gain3/1 -> Scope/1, Sum/1
  Demux2/4 -> Sum13/1, Sum14/2
  Demux2/1 -> Sum15/1, Sum11/2
  Demux2/2 -> Sum13/2, Sum15/2
  Sum12/1 -> Sum11/1
  Sum11/1 -> Gain/1
  Demux2/3 -> Sum12/2, Sum14/1
  Sum13/1 -> Sum12/1
  Input/1 -> Scope1/1, Demux2/1
  Sum/1 -> Demux/1
  Demux/1 -> stateint1/1
  Demux/2 -> stateint2/1
  Demux/3 -> stateint3/1
  Demux/4 -> stateint4/1
  Demux/5 -> stateint5/1
  Demux/6 -> stateint6/1
  Mux1/1 -> states/1
  stateint1/1 -> Mux1/1
  stateint2/1 -> Mux1/2
  stateint3/1 -> Mux1/3
  Sum15/1 -> Scope2/1, Gain1/1
  Sum14/1 -> Gain2/1
  Colored Noise/1 -> Gain3/1
